simulink model "MapControl"  (R2020a)
settings: Solver=ode3  StartTime=0.0  StopTime=10.0  RelTol=1e-3
PreLoadFcn:
  | % Lidar parameters
  | 
  | 
  | scanAngles = linspace(-pi/2,pi/2,360);
  | scanMaxRange = 3.5;
  | scanSensorOffset = [0,0];
model workspace (MAT data in the model file):
  destX = 2
  destY = 2
undefined symbols (not defined in the file or in its folder): Angular, Linear
libraries: robotlib x4, robotcorelib x1
settings Model: Creator=Pierre  LastModifiedBy=pierre
settings OptimizationCC: EnhancedBackFolding=on  PassReuseOutputArgsAs=Individual arguments  ZeroExternalMemoryAtStartup=off  ZeroInternalMemoryAtStartup=off  MaxStackSize=64  OptimizeBlockOrder=speed  DifferentSizesBufferReuse=on  OptimizationCustomize=off  EfficientTunableParamExpr=on
settings DebuggingCC: ParameterTunabilityLossMsg=error
settings HardwareCC: ProdBitPerPointer=32  ProdBitPerSizeT=32  ProdBitPerPtrDiffT=32  ProdLargestAtomicFloat=None  ProdIntDivRoundTo=Undefined  ProdEndianess=Unspecified  ProdWordSize=32  ProdHWDeviceType=Generic->Unspecified (assume 32-bit Generic)
settings RTWCC: SystemTargetFile=ert.tlc  HardwareBoard=Robot Operating System (ROS)  TemplateMakefile=ert_default_tmf  Toolchain=Catkin  TargetLang=C++
settings CodeAppCC: ForceParamTrailComments=on  IgnoreCustomStorageClasses=off  OperatorAnnotations=on  SimulinkDataObjDesc=on  SFDataObjDesc=on  InsertBlockDesc=on

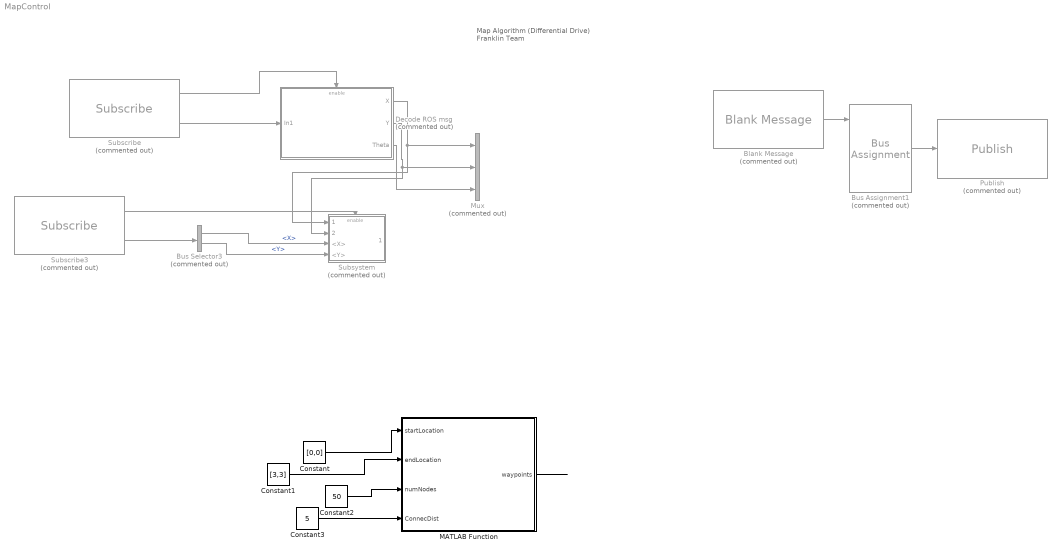
== system MapControl ==
  note: Map Algorithm
      | (Differential Drive)
      |
      | Franklin Team
  Blank Message : robotlib/Blank Message  Commented=on  messageClass=Message  entityType=geometry_msgs/Twist  messageType=geometry_msgs/Twist  SampleTime=inf
  Bus Assignment1 : BusAssignment  Commented=on  AssignedSignals=Linear.X,Angular.Z
  Bus Selector3 : BusSelector  Commented=on  OutputSignals=X,Y
  Constant : Constant  Value=[0,0]
  Constant1 : Constant  Value=[3,3]
  Constant2 : Constant  Value=50
  Constant3 : Constant  Value=5
  Decode ROS msg : Subsystem  Commented=on
  MATLAB Function : MATLAB Function  TreatAsAtomicUnit=on
  Mux : Mux  Commented=on  Inputs=3
  Publish : robotlib/Publish  Commented=on  topicSource=Specify your own  topic=/cmd_vel  messageType=geometry_msgs/Twist  messageQueueLength=1
  Subscribe : robotlib/Subscribe  Commented=on  topicSource=Specify your own  topic=/odom  messageType=nav_msgs/Odometry  sampleTime=-1  messageQueueLength=1
  Subscribe3 : robotlib/Subscribe  Commented=on  topicSource=Specify your own  topic=/destination  messageType=geometry_msgs/Pose2D  sampleTime=1  messageQueueLength=1
  Subsystem : Subsystem  Commented=on
  wires:
  Blank Message/1 -> Bus Assignment1/1
  Bus Assignment1/1 -> Publish/1
  Subscribe3/2 -> Bus Selector3/1
  Subscribe3/1 -> Subsystem/Enable
  Subscribe/2 -> Decode ROS msg/1(In1)
  Subscribe/1 -> Decode ROS msg/Enable
  Decode ROS msg/1(X) -> Subsystem/1(<Xinit>), Mux/1
  Decode ROS msg/2(Y) -> Subsystem/2(<Yinit>), Mux/2
  Decode ROS msg/3(Theta) -> Mux/3
  Bus Selector3/1 -> Subsystem/3(<X>)  "<X>"
  Bus Selector3/2 -> Subsystem/4(<Y>)  "<Y>"
  Constant/1 -> MATLAB Function/1(startLocation)
  Constant1/1 -> MATLAB Function/2(endLocation)
  Constant2/1 -> MATLAB Function/3(numNodes)
  Constant3/1 -> MATLAB Function/4(ConnecDist)
  MATLAB Function/1(waypoints) -> ?

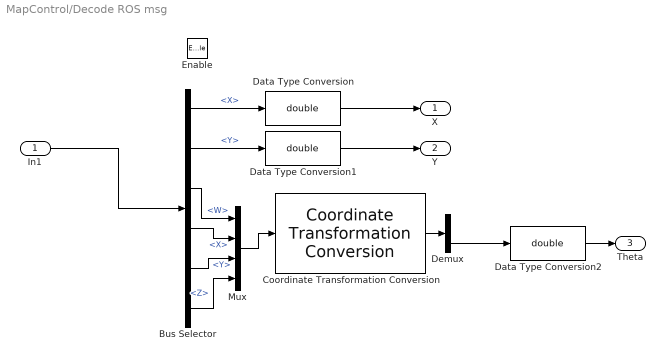
== system MapControl/Decode ROS msg ==
  In1 : Inport
  Enable : EnablePort
  Bus Selector : BusSelector  DialogController=Simulink.DDGSource_BusSelector  OutputSignals=Pose.Pose.Position.X,Pose.Pose.Position.Y,Pose.Pose.Orientation.W,Pose.Pose.Orientation.X,Pose.Pose.Orientation.Y,Pose.Pose.Orientation.Z
  Coordinate Transformation Conversion : robotcorelib/Coordinate Transformation Conversion  InputRepresentation=Quaternion  InputEulerSequence=ZYX  ShowTrVecInputPort=on  OutputRepresentation=Euler Angles  OutputEulerSequence=XYZ  ShowTrVecOutputPort=on  SimulateUsing=Interpreted execution
      settings: SourceProductBaseCode=NV,RO,RR
  Data Type Conversion : DataTypeConversion  OutDataTypeStr=double
  Data Type Conversion1 : DataTypeConversion  OutDataTypeStr=double
  Data Type Conversion2 : DataTypeConversion  OutDataTypeStr=double
  Demux : Demux  Outputs=3
  Mux : Mux
  X : Outport  VectorParamsAs1DForOutWhenUnconnected=off
  Y : Outport  Port=2  VectorParamsAs1DForOutWhenUnconnected=off
  Theta : Outport  Port=3  VectorParamsAs1DForOutWhenUnconnected=off
  wires:
  In1/1 -> Bus Selector/1
  Bus Selector/2 -> Data Type Conversion1/1  "<Y>"
  Bus Selector/1 -> Data Type Conversion/1  "<X>"
  Data Type Conversion/1 -> X/1
  Data Type Conversion1/1 -> Y/1
  Data Type Conversion2/1 -> Theta/1
  Bus Selector/3 -> Mux/1  "<W>"
  Bus Selector/4 -> Mux/2  "<X>"
  Bus Selector/5 -> Mux/3  "<Y>"
  Bus Selector/6 -> Mux/4  "<Z>"
  Mux/1 -> Coordinate Transformation Conversion/1
  Coordinate Transformation Conversion/1 -> Demux/1
  Demux/3 -> Data Type Conversion2/1

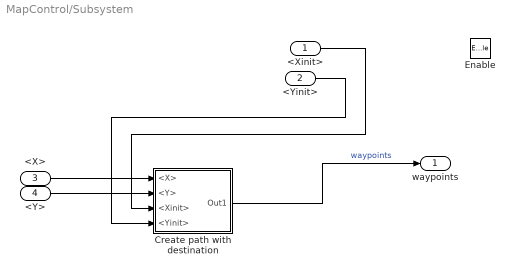
== system MapControl/Subsystem ==
  <Xinit> : Inport
  <Yinit> : Inport  Port=2
  <X> : Inport  Port=3
  <Y> : Inport  Port=4
  Enable : EnablePort
  Create path with destination : Subsystem
  waypoints : Outport
  wires:
  <Yinit>/1 -> Create path with destination/4(<Yinit>)
  <X>/1 -> Create path with destination/1(<X>)
  <Y>/1 -> Create path with destination/2(<Y>)
  Create path with destination/1(Out1) -> waypoints/1  "waypoints"
  <Xinit>/1 -> Create path with destination/3(<Xinit>)

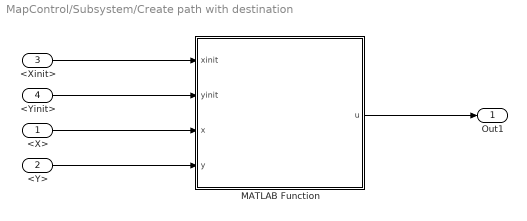
== system MapControl/Subsystem/Create path with destination ==
  <X> : Inport
  <Y> : Inport  Port=2
  <Xinit> : Inport  Port=3
  <Yinit> : Inport  Port=4
  MATLAB Function : MATLAB Function  TreatAsAtomicUnit=on
  Out1 : Outport
  wires:
  <Y>/1 -> MATLAB Function/4(y)
  <X>/1 -> MATLAB Function/3(x)
  MATLAB Function/1(u) -> Out1/1
  <Xinit>/1 -> MATLAB Function/1(xinit)
  <Yinit>/1 -> MATLAB Function/2(yinit)

== matlab function MapControl/Subsystem/Create path with destination/MATLAB Function ==
  data: xinit input; yinit input; x input; y input; u output
function u = newDest(xinit, yinit, x, y)
u = [xinit,yinit; x,y];

== matlab function MapControl/MATLAB Function ==
  data: waypoints output; startLocation input; endLocation input; numNodes input; ConnecDist input
%% numNodes: 
% Define the number of PRM nodes to be used during PRM construction. 
% PRM constructs a roadmap using a given number of nodes on the given map. 
% Based on the dimension and the complexity of the input map, 
% this is one of the primary attributes to tune in order to get a 
% solution between two points on the map. A large number of nodes create 
% a dense roadmap and increases the probability of finding a path. 
% However, having more nodes increases the computation time for both creating 
% the roadmap and finding a solution.
%---------------------
%% ConnecDist: 
% Define the maximum allowed distance between two connected nodes on the map. 
% PRM connects all nodes separated by this distance (or less) on the map. 
% This is another attribute to tune in the case of larger and/or complicated 
% input maps. A large connection distance increases the connectivity between 
% nodes to find a path easier, but can increase the computation time of roadmap creation.

function waypoints = readMapGetPath(startLocation, endLocation, numNodes, ConnecDist)
map = load("map.mat");

%Read the map ...from ROS msg... sh!t
imageNorm = double(map)/255;
imageOccupancy = 1 - imageNorm;
mapi = occupancyMap(imageOccupancy,20);

%Ajust the size to the robot diameter
mapInflated = copy(mapi);
robotRadius = 0.2;
inflate(mapInflated,robotRadius);

%Create a probalistic road map
prm = mobileRobotPRM;
prm.Map = mapInflated;
prm.NumNodes = numNodes;
prm.ConnectionDistance = ConnecDist;

%Find a path (path being probabilistic)
waypoints = findpath(prm, startLocation, endLocation);
